simulink model "test_detection_simulink"  (R2015a)
settings: Solver=ode45  StartTime=0.0  StopTime=inf  RelTol=1e-3
values from neighbouring files (symbols this model uses):
  ReferenceImage = imresize (ReferenceFrame,0.65,'bilinear')    [referenceImage_script.m]
undefined symbols (not defined in the file or in its folder): IsPositionTracked, IsSkeletonTracked, JointDepthIndices, JointImageIndices, JointTrackingState, JointWorldCoordinates, none, PositionDepthIndices, PositionImageIndices, PositionWorldCoordinates, SegmentationData, SkeletonTrackingID, videoinput
libraries: imaqlib x1, visionsinks x1
settings Model: Creator=tzwijger  LastModifiedBy=tzwijger

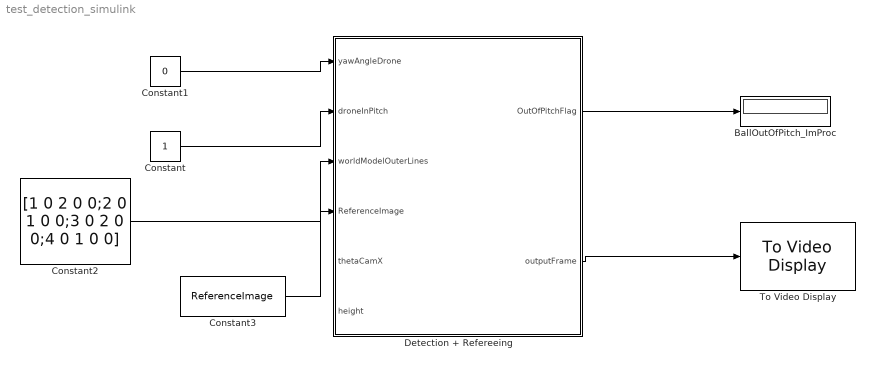
== system test_detection_simulink ==
  BallOutOfPitch_ImProc : Display
  Constant : Constant
  Constant1 : Constant  Value=0
  Constant2 : Constant  Value=[1 0 2 0 0;2 0 1 0 0;3 0 2 0 0;4 0 1 0 0]
  Constant3 : Constant  Value=ReferenceImage
  Detection + Refereeing : Subsystem
  To Video Display : visionsinks/To Video Display  windowSizeMode=True size (1:1)  openAtMdlStart=on  fullScreen=off  videoWindowX=53  videoWindowY=70  saveWindowSize=off  videoWindowWidth=416  videoWindowHeight=312  inputColorFormat=RGB  inputType=Obsolete  imagePorts=One multidimensional signal  OutputDevice=On-screen video monitor  dataOrg=Column-major  isWindowOpen=off
  wires:
  Constant/1 -> Detection + Refereeing/2(droneInPitch)
  Constant1/1 -> Detection + Refereeing/1(yawAngleDrone)
  Constant2/1 -> Detection + Refereeing/3(worldModelOuterLines)
  Detection + Refereeing/1(OutOfPitchFlag) -> BallOutOfPitch_ImProc/1
  Detection + Refereeing/2(outputFrame) -> To Video Display/1
  Constant3/1 -> Detection + Refereeing/4(ReferenceImage)

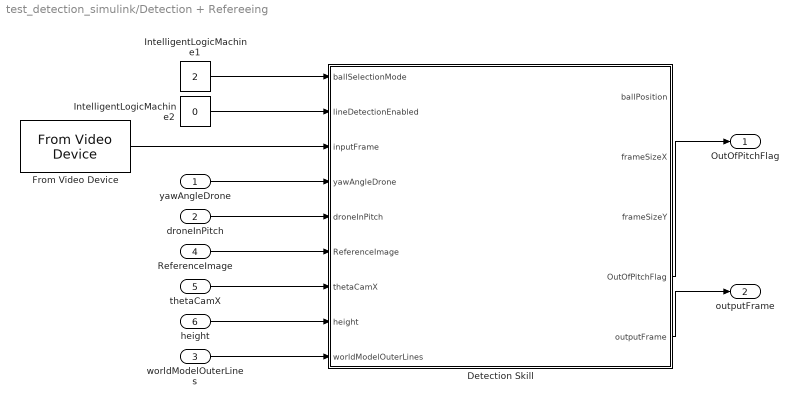
== system test_detection_simulink/Detection + Refereeing ==
  yawAngleDrone : Inport
  droneInPitch : Inport  Port=2
  worldModelOuterLines : Inport  Port=3
  ReferenceImage : Inport  Port=4
  thetaCamX : Inport  Port=5
  height : Inport  Port=6
  Detection Skill : MATLAB Function  TreatAsAtomicUnit=on
  From Video Device : imaqlib/From Video Device  DeviceMenu=winvideo 1 (HP HD Webcam)  Device=winvideo 2 (Logitech HD Webcam C525)  ObjConstructor=videoinput('winvideo', 2)  VideoFormatMenu=RGB24_640x480  VideoFormat=RGB24_640x480  VideoSource=input1  ROIPosition=[0 0 480 640]  EnableHWTrigger=off  TriggerConfiguration=none/none  SampleTime=1/30  OutputPortsMode=One multidimensional signal  DataType=double  CanDoHWTrigger=no  ReturnedColorSpace=rgb  BlockHandle=56.0001  ROIWidth=640  ROIHeight=480  ROIColumn=0  ROIRow=0  EngXMLPath=C:\Program Files\MATLAB\R2015a\toolbox\imaq\imaq\private  DevXMLPath=C:\MATLAB\SupportPackages\R2015a\osgenericvideointerface\toolbox\imaq\supportpackages\genericvideo\adaptor\win64  EngLibPath=C:\Program Files\MATLAB\R2015a\toolbox\imaq\imaqblks\imaqmex\win64  ColorSpace=rgb  BayerSensorAlignment=grbg  AllMetadata=IsPositionTracked;IsSkeletonTracked;JointDepthIndices;JointImageIndices;JointTrackingState;JointWorldCoordinates;PositionDepthIndices;PositionImageIndices;PositionWorldCoordinates;SegmentationData;SkeletonTrackingID
  IntelligentLogicMachine1 : Constant  Value=2
  IntelligentLogicMachine2 : Constant  Value=0
  OutOfPitchFlag : Outport
  outputFrame : Outport  Port=2
  wires:
  Detection Skill/4(OutOfPitchFlag) -> OutOfPitchFlag/1
  Detection Skill/5(outputFrame) -> outputFrame/1
  yawAngleDrone/1 -> Detection Skill/4(yawAngleDrone)
  droneInPitch/1 -> Detection Skill/5(droneInPitch)
  worldModelOuterLines/1 -> Detection Skill/9(worldModelOuterLines)
  IntelligentLogicMachine2/1 -> Detection Skill/2(lineDetectionEnabled)
  From Video Device/1 -> Detection Skill/3(inputFrame)
  IntelligentLogicMachine1/1 -> Detection Skill/1(ballSelectionMode)
  ReferenceImage/1 -> Detection Skill/6(ReferenceImage)
  height/1 -> Detection Skill/8(height)
  thetaCamX/1 -> Detection Skill/7(thetaCamX)

== matlab function test_detection_simulink/Detection + Refereeing/Detection Skill ==
  data: ballPosition output; frameSizeX output; frameSizeY output; ballSelectionMode input; OutOfPitchFlag output; lineDetectionEnabled input; inputFrame input; yawAngleDrone input; droneInPitch input; ReferenceImage input; thetaCamX input; height input; worldModelOuterLines input; outputFrame output


function [ballPosition,...
          frameSizeX,...
          frameSizeY,...
          OutOfPitchFlag,...
          outputFrame]  = detectionSkillAndRefereeing(ballSelectionMode,... 
                                                      lineDetectionEnabled,... 
                                                      inputFrame,...
                                                      yawAngleDrone,...
                                                      droneInPitch,...
                                                      ReferenceImage,...
                                                      thetaCamX,...
                                                      height,...
                                                      worldModelOuterLines)
                                                 
    coder.extrinsic('detectionSkill','refereeingOutOfPitch')
    
     % Prepare outputs detection skill
     ballPosition = zeros(1,2);
%     selectedLines = zeros(50,2);
%      ballStatusFlag = 0;
%      lineStatusFlag = 0;
     outputFrame = zeros([240 320 3]);
    
    % Prepare outputs Refereeing function
    OutOfPitchFlag = 0;
    
    % Prepare constant/unused inputs Refereeing function
    lineWidth = 0;
    frameProperties = size(inputFrame);
    numOutOfBoundLines = sum(worldModelOuterLines(:,2));
    
    
    [ballPosition,... 
     selectedLines,... 
     outputFrame] = detectionSkill(ballSelectionMode,... 
                                   lineDetectionEnabled,...
                                   ReferenceImage,...
                                   inputFrame);
    
    OutOfPitchFlag  = refereeingOutOfPitch(yawAngleDrone,...
                                           ballPosition,...
                                           lineWidth,...
                                           selectedLines,...
                                           numOutOfBoundLines,...
                                           frameProperties,...
                                           droneInPitch,...
                                           thetaCamX,...
                                           height,...                                           
                                           worldModelOuterLines);
end
